simulink model "MRAMR_SIMULINK"  (R2023a)
settings: Solver=VariableStepAuto  StartTime=0.0  StopTime=10.0  RelTol=1e-3
values from neighbouring files (symbols this model uses):
  b1 = 1000    [MRAMR.m]    (also in c_MRAMR_SIMULINK.m)
  k1 = 16182    [MRAMR.m]    (also in c_MRAMR_SIMULINK.m)
  k2 = 19000    [MRAMR.m]    (also in c_MRAMR_SIMULINK.m)
  m1 = 290    [MRAMR.m]    (also in c_MRAMR_SIMULINK.m)
  m2 = 59    [MRAMR.m]    (also in c_MRAMR_SIMULINK.m)
settings Model: Creator=Pablo  LastModifiedBy=Pablo

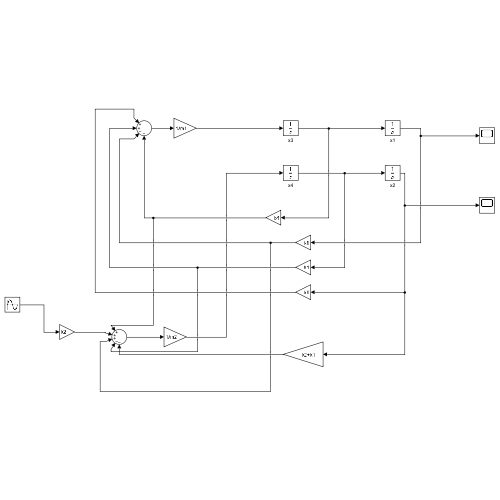
[thumbnail: Simulink's stored preview of the top-level diagram]
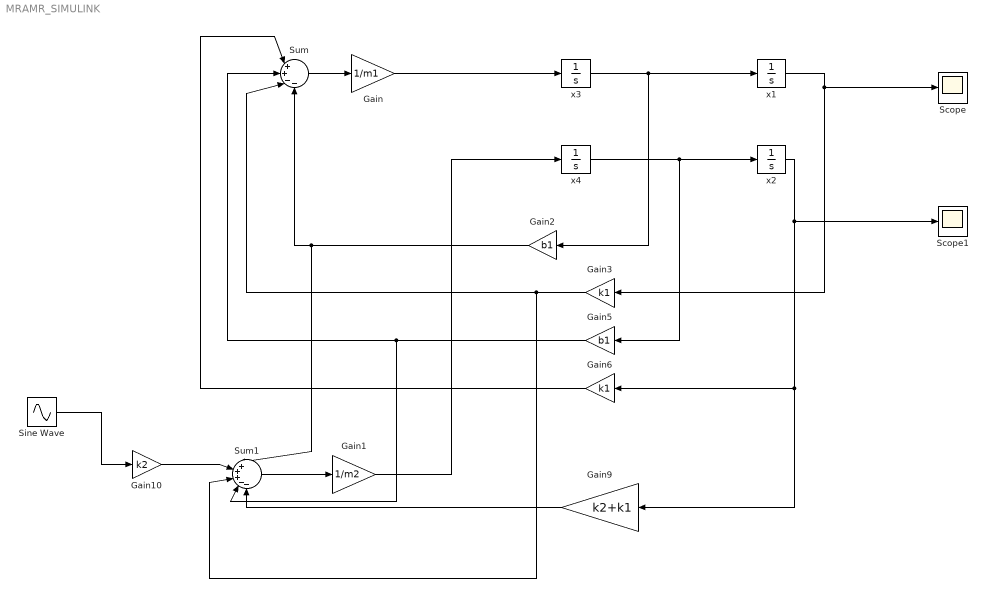
== system MRAMR_SIMULINK ==
  Gain : Gain  Gain=1/m1
  Gain1 : Gain  Gain=1/m2
  Gain10 : Gain  Gain=k2
  Gain2 : Gain  Gain=b1
  Gain3 : Gain  Gain=k1
  Gain5 : Gain  Gain=b1
  Gain6 : Gain  Gain=k1
  Gain9 : Gain  Gain=k2+k1
  Scope : Scope
  Scope1 : Scope
  Sine Wave : Sin  Amplitude=.05  Frequency=.5*pi  SampleTime=0
  Sum : Sum  Inputs=|++--
  Sum1 : Sum  Inputs=|+++--
  x{1..4} (4 alike) : Integrator
  wires:
  Sum/1 -> Gain/1
  Gain5/1 -> Sum1/4, Sum/2
  x1/1 -> Gain3/1, Scope/1
  x2/1 -> Scope1/1, Gain9/1, Gain6/1
  Gain6/1 -> Sum/1
  Gain9/1 -> Sum1/5
  Gain3/1 -> Sum1/3, Sum/3
  Gain2/1 -> Sum/4, Sum1/1
  Sum1/1 -> Gain1/1
  Gain/1 -> x3/1
  x4/1 -> Gain5/1, x2/1
  x3/1 -> x1/1, Gain2/1
  Gain1/1 -> x4/1
  Sine Wave/1 -> Gain10/1
  Gain10/1 -> Sum1/2
